simulink model "el_pr"  (R2022b)
settings: Solver=VariableStepAuto  StartTime=0.0  StopTime=13  RelTol=1e-3
values from neighbouring files (symbols this model uses):
  alpha_trim = (((Cz_trim + Cz_alp*alpha_0)*(-1*Cm_delm)/Cz_delm) - Cm_0 + (alpha_0*Cm_alpha))/(Cm_alpha + (Cz_alp*(-1*Cm_delm)/Cz_delm))    [variableLoader.m]
  delt_trim = sqrt((T_trim/(ro*Sprop*Cprop/(2*m))) + velocity*velocity)/kMotor    [variableLoader.m]
  delta_m_trim = ((alpha_trim - alpha_0)*Cm_alpha + Cm_0)/(-1*Cm_delm)    [variableLoader.m]
  velocity = 25    [variableLoader.m]

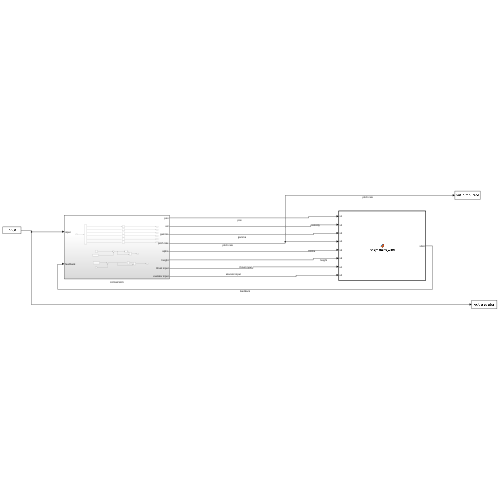
[thumbnail: Simulink's stored preview of the top-level diagram]
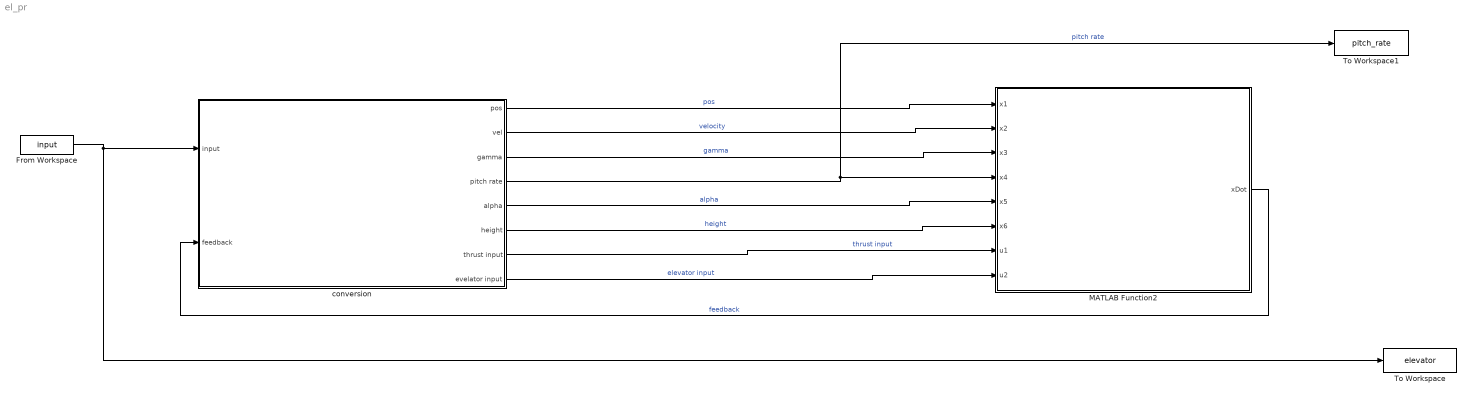
== system el_pr ==
  From Workspace : FromWorkspace  VariableName=input  SampleTime=0.02
  MATLAB Function2 : MATLAB Function  TreatAsAtomicUnit=on
  To Workspace : ToWorkspace  VariableName=elevator  SampleTime=0.02
  To Workspace1 : ToWorkspace  VariableName=pitch_rate  SampleTime=0.02
  conversion : Subsystem
  wires:
  conversion/5(alpha) -> MATLAB Function2/5(x5)  "alpha"
  conversion/2(vel) -> MATLAB Function2/2(x2)  "velocity"
  conversion/1(pos) -> MATLAB Function2/1(x1)  "pos"
  conversion/6(height) -> MATLAB Function2/6(x6)  "height"
  conversion/3(gamma) -> MATLAB Function2/3(x3)  "gamma"
  conversion/7(thrust input) -> MATLAB Function2/7(u1)  "thrust input"
  conversion/8(evelator input) -> MATLAB Function2/8(u2)  "elevator input"
  MATLAB Function2/1(xDot) -> conversion/2(feedback)  "feedback"
  From Workspace/1 -> conversion/1(input), To Workspace/1
  conversion/4(pitch rate) -> To Workspace1/1, MATLAB Function2/4(x4)  "pitch rate"

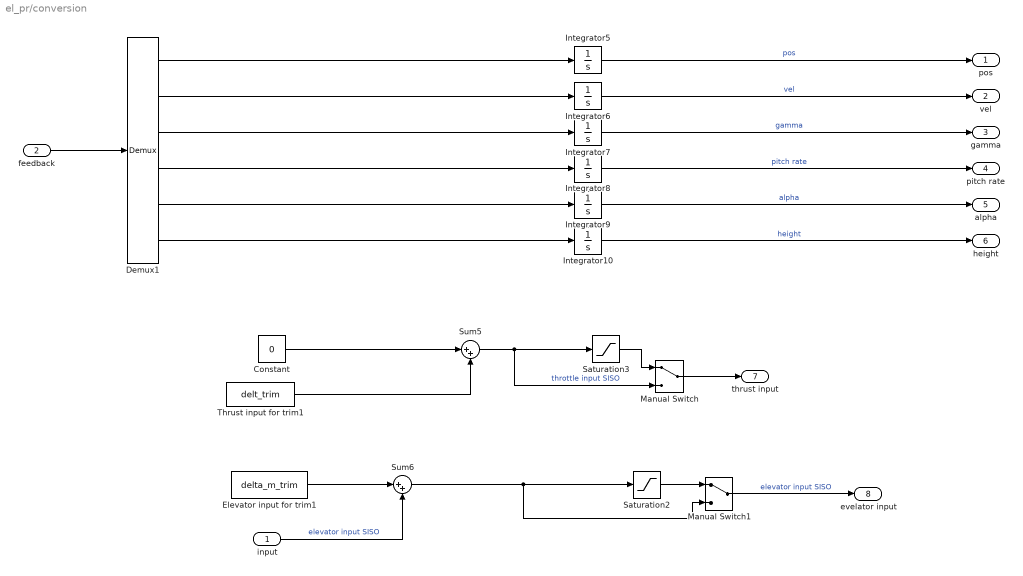
== system el_pr/conversion ==
  input : Inport
  feedback : Inport  Port=2
  Constant : Constant  Value=0
  Demux1 : Demux  Outputs=6
  Elevator input for trim1 : Constant  Value=delta_m_trim
  Integrator10 : Integrator  InitialCondition=50
  Integrator5 : Integrator
  Integrator6 : Integrator  InitialCondition=velocity
  Integrator7 : Integrator
  Integrator8 : Integrator
  Integrator9 : Integrator  InitialCondition=alpha_trim
  Manual Switch : ManualSwitch
  Manual Switch1 : ManualSwitch
  Saturation2 : Saturate  UpperLimit=deg2rad(30)  LowerLimit=-deg2rad(30)
  Saturation3 : Saturate  UpperLimit=1  LowerLimit=0
  Sum5 : Sum  Inputs=|++
  Sum6 : Sum  Inputs=|++
  Thrust input for trim1 : Constant  Value=delt_trim
  pos : Outport
  vel : Outport  Port=2
  gamma : Outport  Port=3
  pitch rate : Outport  Port=4
  alpha : Outport  Port=5
  height : Outport  Port=6
  thrust input : Outport  Port=7
  evelator input : Outport  Port=8
  wires:
  Demux1/4 -> Integrator8/1
  Demux1/3 -> Integrator7/1
  Demux1/2 -> Integrator6/1
  Demux1/5 -> Integrator9/1
  Demux1/6 -> Integrator10/1
  Demux1/1 -> Integrator5/1
  Integrator10/1 -> height/1  "height"
  Integrator7/1 -> gamma/1  "gamma"
  Integrator9/1 -> alpha/1  "alpha"
  Integrator8/1 -> pitch rate/1  "pitch rate"
  Integrator5/1 -> pos/1  "pos"
  Integrator6/1 -> vel/1  "vel"
  feedback/1 -> Demux1/1
  input/1 -> Sum6/2  "elevator input SISO"
  Saturation3/1 -> Manual Switch/1
  Thrust input for trim1/1 -> Sum5/2
  Saturation2/1 -> Manual Switch1/1
  Sum6/1 -> Saturation2/1, Manual Switch1/2
  Manual Switch1/1 -> evelator input/1  "elevator input SISO"
  Sum5/1 -> Manual Switch/2, Saturation3/1  "throttle input SISO"
  Elevator input for trim1/1 -> Sum6/1
  Manual Switch/1 -> thrust input/1
  Constant/1 -> Sum5/1

== matlab function el_pr/MATLAB Function2 ==
function xDot = acDynamics_wind(x1,x2,x3,x4,x5,x6,u1,u2)
    
    Cz_alp = 3.45;
    alpha_0 = 0.4712;
    Cz_delm = -0.36;
    Cx_0 = 0.03;
    %ki = 0.055;
    Cm_0 = -0.02338;
    Cm_alpha = -0.38;
    Cm_q = -3.6;
    L = 0.18994;
    Cm_delm = -0.5;
    S = 0.55;
    B = 1.135;
    m = 13.5;
    Sprop = 0.2027;
    ro = 1.2682;
    kMotor = 80;
    Cprop = 1;
    g = 9.8;
    % A/c DYNAMICS
    p = x1;
    V = x2;
    gamma = x3;
    q = x4;
    alpha = x5;
    h = x6;
    dt = u1;
    delm = u2;
    ki = 0.18994/(pi*2.8956*0.1592);
    T = (ro*Sprop*Cprop/(2*m))*((kMotor*dt)^2 - V*V);
    velocity = 25;
    Cz_trim= m*g*cos(0)/(0.5*ro*velocity*velocity*S);
    alpha_trim = (((Cz_trim + Cz_alp*alpha_0)*(-1*Cm_delm)/Cz_delm) - Cm_0 + (alpha_0*Cm_alpha))/(Cm_alpha + (Cz_alp*(-1*Cm_delm)/Cz_delm));
    delta_m_trim = ((alpha_trim - alpha_0)*Cm_alpha + Cm_0)/(-1*Cm_delm);
    Cz_trim = Cz_alp*(alpha_trim - alpha_0) + Cz_delm*delta_m_trim;
    Cx_trim = Cx_0 + ki*Cz_trim^2;
    T_trim =  0.5*ro*velocity*velocity*S*(Cx_trim);

    Cz = Cz_alp*(alpha - alpha_0) + Cz_delm*delm;
    Cx = Cx_0 + ki*Cz^2;
    Cm_G = Cm_0 + Cm_alpha*(alpha - alpha_0) + Cm_q*q*L/V + Cm_delm*delm;
    p_dot = V*cos(gamma); 
    V_dot = (-m*g*sin(gamma) - 0.5*ro*V*V*S*(Cx) + T)/m;
    %V_dot = 0;
    gamma_dot = (m*g*cos(gamma) - 0.5*ro*V*V*S*Cz)/(-m*V);
    
    q_dot = 0.5*ro*V*V*S*L*Cm_G/B;
    
    alpha_dot = q - gamma_dot;
    
    h_dot = V*sin(gamma);
    xDot = [p_dot V_dot gamma_dot q_dot alpha_dot h_dot];
end
